simulink library "ROS_lib"  (R2019a)
settings: Solver=VariableStepAuto  StartTime=0.0  StopTime=10.0  RelTol=1e-3
undefined symbols (not defined in the file or in its folder): DiscIntNeverNeededParam
libraries: adeye_lib x26, robotlib x4, PreScanSimulinkLibrary x3
settings Model: Creator=adeye  LastModifiedBy=adeye

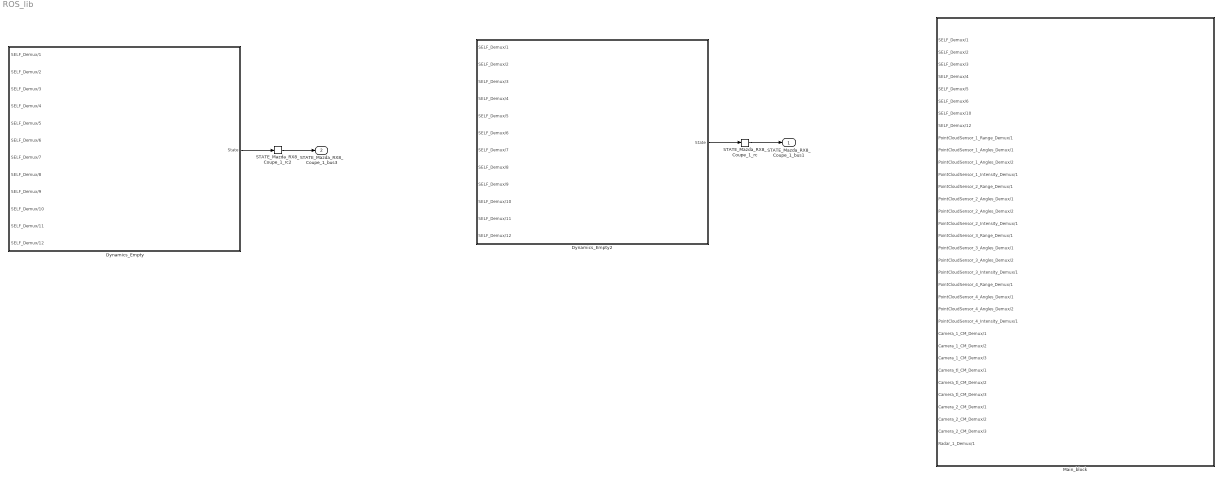
== system ROS_lib ==
  Dynamics_Empty : Subsystem  Tag=Dynamics_Empty
  Dynamics_Empty2 : Subsystem  Tag=Dynamics_Empty
  Main_block : Subsystem
  STATE_Mazda_RX8_Coupe_1_rc : RateTransition  Tag=mux_rc/StatePort  OutPortSampleTimeOpt=Inherit
  STATE_Mazda_RX8_Coupe_1_rc2 : RateTransition  Tag=mux_rc/StatePort  OutPortSampleTimeOpt=Inherit
  STATE_Mazda_RX8_Coupe_1_bus1 : Outport  Tag=outport/StatePort  OutDataTypeStr=Bus: PRESCAN_STATEACTUATORDATA  PortDimensions=1  SampleTime=1/20
  STATE_Mazda_RX8_Coupe_1_bus3 : Outport  Tag=outport/StatePort  Port=2  OutDataTypeStr=Bus: PRESCAN_STATEACTUATORDATA  PortDimensions=1  SampleTime=1/20
  wires:
  STATE_Mazda_RX8_Coupe_1_rc/1 -> STATE_Mazda_RX8_Coupe_1_bus1/1
  Dynamics_Empty2/1(State) -> STATE_Mazda_RX8_Coupe_1_rc/1
  STATE_Mazda_RX8_Coupe_1_rc2/1 -> STATE_Mazda_RX8_Coupe_1_bus3/1
  Dynamics_Empty/1(State) -> STATE_Mazda_RX8_Coupe_1_rc2/1

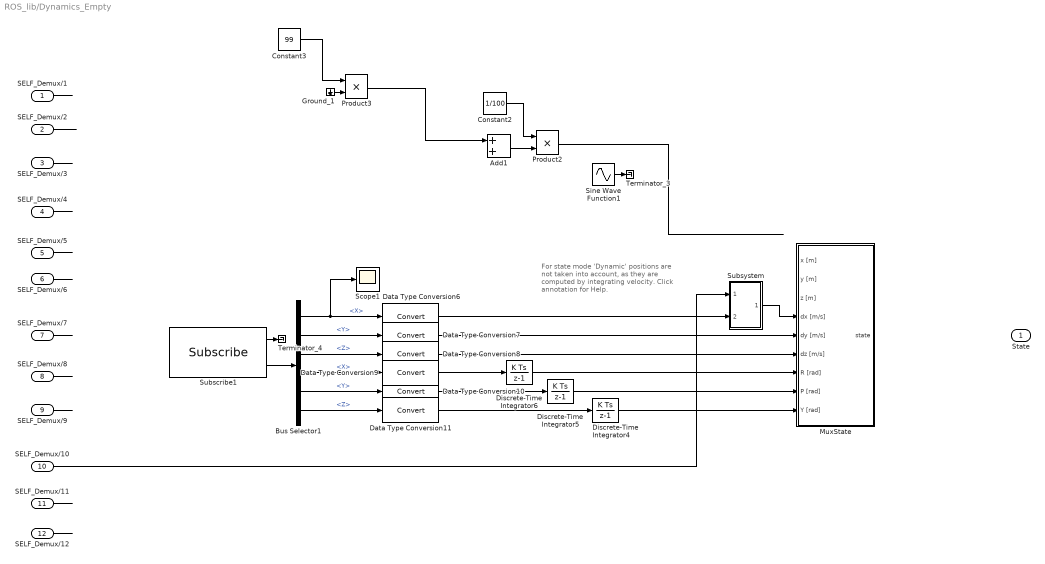
== system ROS_lib/Dynamics_Empty ==
  note: For state mode 'Dynamic' positions
      | are not taken into account, as they
      | are computed by integrating velocity.
      | Click annotation for Help.
  SELF_Demux/1 : Inport
  SELF_Demux/2 : Inport  Port=2
  SELF_Demux/3 : Inport  Port=3
  SELF_Demux/4 : Inport  Port=4
  SELF_Demux/5 : Inport  Port=5
  SELF_Demux/6 : Inport  Port=6
  SELF_Demux/7 : Inport  Port=7
  SELF_Demux/8 : Inport  Port=8
  SELF_Demux/9 : Inport  Port=9
  SELF_Demux/10 : Inport  Port=10
  SELF_Demux/11 : Inport  Port=11
  SELF_Demux/12 : Inport  Port=12
  Add1 : Sum
  Bus Selector1 : BusSelector  OutputSignals=Twist.Linear.X,Twist.Linear.Y,Twist.Linear.Z,Twist.Angular.X,Twist.Angular.Y,Twist.Angular.Z
  Constant2 : Constant  Value=1/100
  Constant3 : Constant  Value=99
  Data Type Conversion{6..11} (6 alike) : DataTypeConversion
  Discrete-Time Integrator4 : DiscreteIntegrator  SampleTime=-1  ICPrevOutput=DiscIntNeverNeededParam  ICPrevScaledInput=DiscIntNeverNeededParam
  Discrete-Time Integrator5 : DiscreteIntegrator  SampleTime=-1  ICPrevOutput=DiscIntNeverNeededParam  ICPrevScaledInput=DiscIntNeverNeededParam
  Discrete-Time Integrator6 : DiscreteIntegrator  SampleTime=-1  ICPrevOutput=DiscIntNeverNeededParam  ICPrevScaledInput=DiscIntNeverNeededParam
  Ground_1 : Ground
  MuxState : Subsystem  Tag=mux/State  mask(Empty Dynamics State Block){positioningmode=off, TimeStep=1/20}
      mask prompts: positioningmode "Positioning Mode"; TimeStep "Auto Assigned: Time Step [s]"
      mask help:
      | Build the state of an actor based on user input.
      | The user can either use positioning mode or dynamics mode.
      | - When using positioning mode the position and orientation of the actor are set directly based on the input. Expected input is relative to the initial position and orientation of the actor. It's also possible to specify the velocity of the actor, though this input isn't used, only passed on.
      | - When using dynamics mode the position input is ignored. Expected input is velocity and orientation. The velocity is relative the current orientation of the actor, while orientation is relative to its initial orientation. The position of the actor is calculated based on the velocity and orientation given.
      settings: DeleteFcn=PreScanBlockDeleteFcn;
  Product2 : Product
  Product3 : Product
  Scope1 : Scope
  Sine Wave Function1 : Sin  Amplitude=0.1  SampleTime=0
  Subscribe1 : robotlib/Subscribe  topicSource=Select from ROS network  topic=/TwistS  messageType=geometry_msgs/TwistStamped  sampleTime=-1  messageQueueLength=1
      settings: SourceProductBaseCode=RO
  Subsystem : Subsystem
  Terminator_3 : Terminator
  Terminator_4 : Terminator
  State : Outport  Tag=outport/StateOutport  SampleTime=1/20
  wires:
  SELF_Demux/1/1 -> ?
  SELF_Demux/2/1 -> ?
  SELF_Demux/12/1 -> ?
  SELF_Demux/6/1 -> ?
  SELF_Demux/11/1 -> ?
  SELF_Demux/8/1 -> ?
  SELF_Demux/9/1 -> ?
  SELF_Demux/7/1 -> ?
  SELF_Demux/4/1 -> ?
  SELF_Demux/3/1 -> ?
  SELF_Demux/5/1 -> ?
  Product2/1 -> ?
  ? -> Add1/2
  Add1/1 -> Product2/2
  Constant2/1 -> Product2/1
  Bus Selector1/5 -> Data Type Conversion10/1  "<Y>"
  Sine Wave Function1/1 -> Terminator_3/1
  Data Type Conversion6/1 -> Subsystem/2(In2)
  Subsystem/1(Out1) -> MuxState/4(dx [m/s])
  Data Type Conversion9/1 -> Discrete-Time Integrator6/1
  Ground_1/1 -> Product3/2
  Subscribe1/1 -> Terminator_4/1
  Subscribe1/2 -> Bus Selector1/1
  Bus Selector1/4 -> Data Type Conversion9/1  "<X>"
  Product3/1 -> Add1/1
  Data Type Conversion11/1 -> Discrete-Time Integrator4/1
  Discrete-Time Integrator4/1 -> MuxState/9(Y [rad])
  Discrete-Time Integrator6/1 -> MuxState/7(R [rad])
  Data Type Conversion8/1 -> MuxState/6(dz [m/s])
  Data Type Conversion10/1 -> Discrete-Time Integrator5/1
  Data Type Conversion7/1 -> MuxState/5(dy [m/s])
  SELF_Demux/10/1 -> Subsystem/1(In1)
  Bus Selector1/1 -> Scope1/1, Data Type Conversion6/1  "<X>"
  Bus Selector1/3 -> Data Type Conversion8/1  "<Z>"
  Discrete-Time Integrator5/1 -> MuxState/8(P [rad])
  Constant3/1 -> Product3/1
  Bus Selector1/6 -> Data Type Conversion11/1  "<Z>"
  Bus Selector1/2 -> Data Type Conversion7/1  "<Y>"

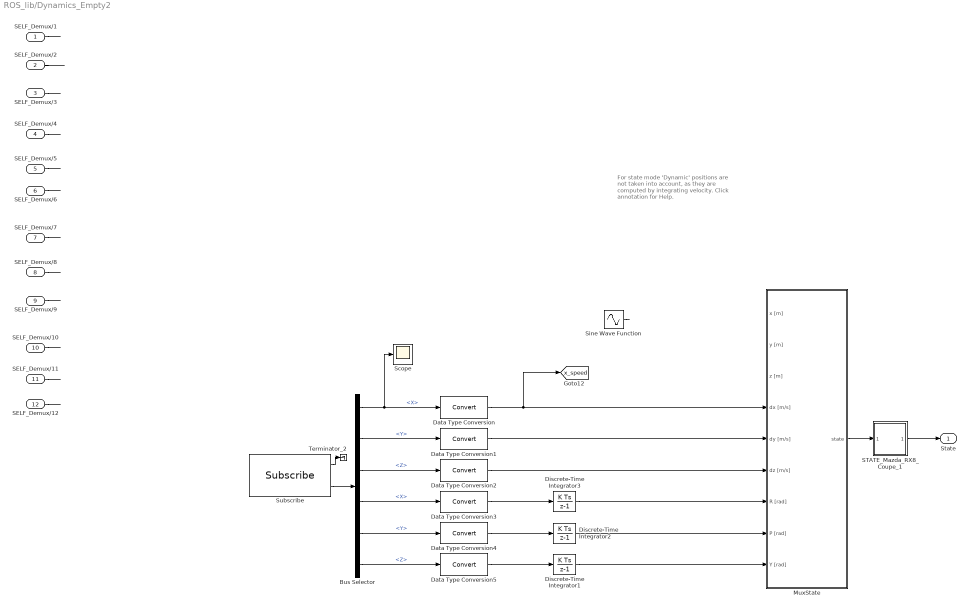
== system ROS_lib/Dynamics_Empty2 ==
  note: For state mode 'Dynamic' positions
      | are not taken into account, as they
      | are computed by integrating velocity.
      | Click annotation for Help.
  SELF_Demux/1 : Inport
  SELF_Demux/2 : Inport  Port=2
  SELF_Demux/3 : Inport  Port=3
  SELF_Demux/4 : Inport  Port=4
  SELF_Demux/5 : Inport  Port=5
  SELF_Demux/6 : Inport  Port=6
  SELF_Demux/7 : Inport  Port=7
  SELF_Demux/8 : Inport  Port=8
  SELF_Demux/9 : Inport  Port=9
  SELF_Demux/10 : Inport  Port=10
  SELF_Demux/11 : Inport  Port=11
  SELF_Demux/12 : Inport  Port=12
  Bus Selector : BusSelector  OutputSignals=Twist.Linear.X,Twist.Linear.Y,Twist.Linear.Z,Twist.Angular.X,Twist.Angular.Y,Twist.Angular.Z
  Data Type Conversion{,1..5} (6 alike) : DataTypeConversion
  Discrete-Time Integrator1 : DiscreteIntegrator  SampleTime=-1  ICPrevOutput=DiscIntNeverNeededParam  ICPrevScaledInput=DiscIntNeverNeededParam
  Discrete-Time Integrator2 : DiscreteIntegrator  SampleTime=-1  ICPrevOutput=DiscIntNeverNeededParam  ICPrevScaledInput=DiscIntNeverNeededParam
  Discrete-Time Integrator3 : DiscreteIntegrator  SampleTime=-1  ICPrevOutput=DiscIntNeverNeededParam  ICPrevScaledInput=DiscIntNeverNeededParam
  MuxState : Subsystem  Tag=mux/State  mask(Empty Dynamics State Block){positioningmode=off, TimeStep=1/20}
      mask prompts: positioningmode "Positioning Mode"; TimeStep "Auto Assigned: Time Step [s]"
      mask help:
      | Build the state of an actor based on user input.
      | The user can either use positioning mode or dynamics mode.
      | - When using positioning mode the position and orientation of the actor are set directly based on the input. Expected input is relative to the initial position and orientation of the actor. It's also possible to specify the velocity of the actor, though this input isn't used, only passed on.
      | - When using dynamics mode the position input is ignored. Expected input is velocity and orientation. The velocity is relative the current orientation of the actor, while orientation is relative to its initial orientation. The position of the actor is calculated based on the velocity and orientation given.
      settings: DeleteFcn=PreScanBlockDeleteFcn;
  STATE_Mazda_RX8_Coupe_1 : Subsystem  Tag=mux/StatePort  Priority=0  LoadFcn=load PrescanStateActuatorData  mask(PreScan Sink Block: State){x0=74.1475, y0=27.5553, z0=0.51, Roll0=0, Pitch0=0, Yaw0=0, TimeStep=1/20}
      mask prompts: x0 "Ini x-position VEHICLE wrt GLOBAL axis system [m]"; y0 "Ini y-position VEHICLE wrt GLOBAL axis system [m]"; z0 "Ini z-position VEHICLE wrt GLOBAL axis system [m]"; Roll0 "Ini roll-angle BODY wrt VEHICLE axis system [deg]"; Pitch0 "Ini pitch-angle BODY wrt VEHICLE axis system [deg]"; Yaw0 "Ini yaw-angle VEHICLE wrt GLOBAL axis system [deg]"; TimeStep "Auto-Assigned: Upload Period [s]"
      mask help:
      | The Actor State contains a vector signal of size (9x1), containing the following signals:
      |
      | -  Position                  (x,y,z)                                     [m]
      | -  Velocity                  (vx,vy,vz)                               [m/s]
      | -  Angles                    (Roll, Pitch, Yaw)                   [rad]
      |
      | The Actor state is defined in the global axis system.
      | The state is superponed on the Initial position defined in the GUI.
      |
      | For more information, please click Help.
      settings: DeleteFcn=PreScanBlockDeleteFcn;
      mask Help: eval('openHelp(222)')
      mask Display: image(imread('State.png'))
  Scope : Scope
  Sine Wave Function : Sin  Amplitude=0.1  SampleTime=0
  Subscribe : robotlib/Subscribe  topicSource=Select from ROS network  topic=/TwistS  messageType=geometry_msgs/TwistStamped  sampleTime=-1  messageQueueLength=1
      settings: SourceProductBaseCode=RO
  Terminator_2 : Terminator
  State : Outport  Tag=outport/StateOutport  SampleTime=1/20
  tag scope: x_speed=global
  wires:
  Bus Selector/1 -> Scope/1, Data Type Conversion/1  "<X>"
  Data Type Conversion/1 -> [x_speed], MuxState/4(dx [m/s])
  Bus Selector/2 -> Data Type Conversion1/1  "<Y>"
  Bus Selector/3 -> Data Type Conversion2/1  "<Z>"
  Bus Selector/4 -> Data Type Conversion3/1  "<X>"
  Data Type Conversion3/1 -> Discrete-Time Integrator3/1
  Bus Selector/5 -> Data Type Conversion4/1  "<Y>"
  Data Type Conversion4/1 -> Discrete-Time Integrator2/1
  Bus Selector/6 -> Data Type Conversion5/1  "<Z>"
  Data Type Conversion5/1 -> Discrete-Time Integrator1/1
  Subscribe/2 -> Bus Selector/1
  Data Type Conversion1/1 -> MuxState/5(dy [m/s])
  Data Type Conversion2/1 -> MuxState/6(dz [m/s])
  Discrete-Time Integrator3/1 -> MuxState/7(R [rad])
  Discrete-Time Integrator2/1 -> MuxState/8(P [rad])
  Discrete-Time Integrator1/1 -> MuxState/9(Y [rad])
  Sine Wave Function/1 -> ?
  Subscribe/1 -> Terminator_2/1
  MuxState/1(state) -> STATE_Mazda_RX8_Coupe_1/1(State)
  STATE_Mazda_RX8_Coupe_1/1(StateBus) -> State/1
  SELF_Demux/1/1 -> ?
  SELF_Demux/2/1 -> ?
  SELF_Demux/12/1 -> ?
  SELF_Demux/6/1 -> ?
  SELF_Demux/11/1 -> ?
  SELF_Demux/8/1 -> ?
  SELF_Demux/9/1 -> ?
  SELF_Demux/7/1 -> ?
  SELF_Demux/4/1 -> ?
  SELF_Demux/10/1 -> ?
  SELF_Demux/3/1 -> ?
  SELF_Demux/5/1 -> ?

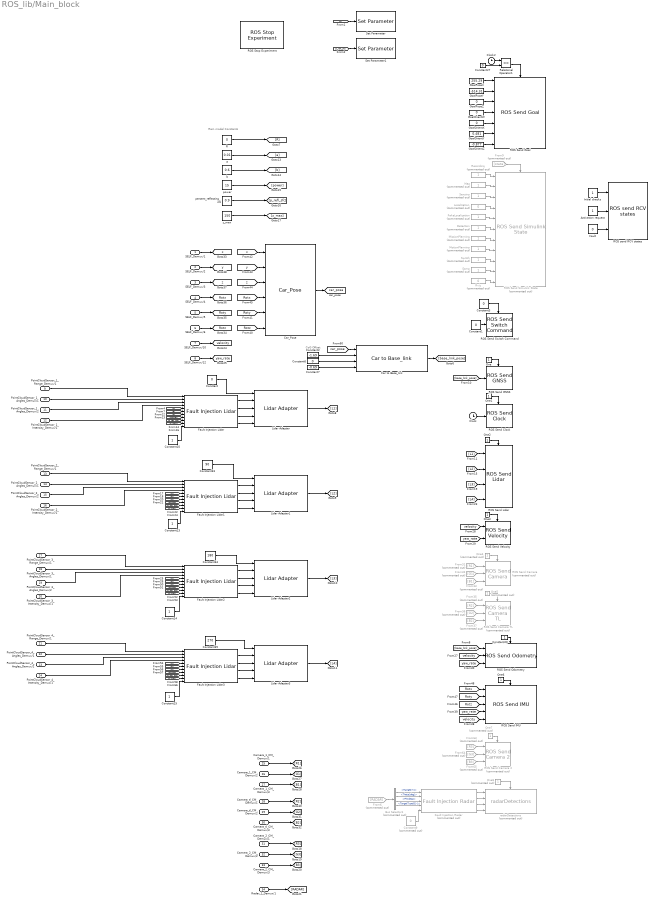
== system ROS_lib/Main_block ==
  note: Rain model Constants
  note: CoG Offset
  SELF_Demux/1 : Inport
  SELF_Demux/2 : Inport  Port=2
  SELF_Demux/3 : Inport  Port=3
  SELF_Demux/4 : Inport  Port=4
  SELF_Demux/5 : Inport  Port=5
  SELF_Demux/6 : Inport  Port=6
  SELF_Demux/10 : Inport  Port=7
  SELF_Demux/12 : Inport  Port=8
  PointCloudSensor_1_Range_Demux/1 : Inport  Port=9
  PointCloudSensor_1_Angles_Demux/1 : Inport  Port=10
  PointCloudSensor_1_Angles_Demux/2 : Inport  Port=11
  PointCloudSensor_1_Intensity_Demux/1 : Inport  Port=12
  PointCloudSensor_2_Range_Demux/1 : Inport  Port=13
  PointCloudSensor_2_Angles_Demux/1 : Inport  Port=14
  PointCloudSensor_2_Angles_Demux/2 : Inport  Port=15
  PointCloudSensor_2_Intensity_Demux/1 : Inport  Port=16
  PointCloudSensor_3_Range_Demux/1 : Inport  Port=17
  PointCloudSensor_3_Angles_Demux/1 : Inport  Port=18
  PointCloudSensor_3_Angles_Demux/2 : Inport  Port=19
  PointCloudSensor_3_Intensity_Demux/1 : Inport  Port=20
  PointCloudSensor_4_Range_Demux/1 : Inport  Port=21
  PointCloudSensor_4_Angles_Demux/1 : Inport  Port=22
  PointCloudSensor_4_Angles_Demux/2 : Inport  Port=23
  PointCloudSensor_4_Intensity_Demux/1 : Inport  Port=24
  Camera_1_CM_Demux/1 : Inport  Port=25
  Camera_1_CM_Demux/2 : Inport  Port=26
  Camera_1_CM_Demux/3 : Inport  Port=27
  Camera_tl_CM_Demux/1 : Inport  Port=28
  Camera_tl_CM_Demux/2 : Inport  Port=29
  Camera_tl_CM_Demux/3 : Inport  Port=30
  Camera_2_CM_Demux/1 : Inport  Port=31
  Camera_2_CM_Demux/2 : Inport  Port=32
  Camera_2_CM_Demux/3 : Inport  Port=33
  Radar_1_Demux/1 : Inport  Port=34
  Activation request : Constant  OutDataTypeStr=Inherit: Inherit via back propagation
  Bus Selector1 : BusSelector  Commented=on  OutputSignals=Range[m],Theta[deg],Phi[deg],TargetTypeID[-]
  Car to Base_link : adeye_lib/Car to Base_link  SystemSampleTime=-1
  Car_Pose : adeye_lib/Car_Pose  SystemSampleTime=-1
  Clock : Clock
  Clock2 : Clock
  Constant : Constant  Value=0  OutDataTypeStr=Inherit: Inherit via back propagation
  Constant1 : Constant  Value=0  OutDataTypeStr=int32
  Constant{10,13..15} (4 alike) : Constant  OutDataTypeStr=Inherit: Inherit via back propagation
  Constant2 : Constant  Value=-1.69
  Constant20 : Constant
  Constant27 : Constant  Value=0
  Constant3 : Constant  Value=0
  Constant33 : Constant  Value=90  OutDataTypeStr=Inherit: Inherit via back propagation
  Constant34 : Constant  Value=180  OutDataTypeStr=Inherit: Inherit via back propagation
  Constant35 : Constant  Value=270  OutDataTypeStr=Inherit: Inherit via back propagation
  Constant6 : Constant  Value=0
  Constant7 : Constant  Value=-0.69
  Constant9 : Constant  Commented=on  Value=0
  Detection : Constant  Commented=on
  FakeLocalization : Constant  Commented=on
  Fault : Constant  Value=0  OutDataTypeStr=Inherit: Inherit via back propagation
  Fault Injection Lidar{,1..3} (4 alike) : adeye_lib/Fault Injection Lidar  vr=0.0001  vi=0.0001  f=20  p=225*16
  Fault Injection Radar : adeye_lib/Fault Injection Radar  Commented=on  n=7  vr=1  vt=1  vp=1
  From31 : From  Commented=on  GotoTag=R1
  From32 : From  Commented=on  GotoTag=G1
  From33 : From  Commented=on  GotoTag=B1
  From35 : From  Commented=on  GotoTag=R2
  From36 : From  Commented=on  GotoTag=G2
  From37 : From  Commented=on  GotoTag=B2
  From6 : From  Commented=on  GotoTag=RADAR
  From63 : From  Commented=on  GotoTag=R3
  From64 : From  Commented=on  GotoTag=G3
  From65 : From  Commented=on  GotoTag=B3
  From9 : From  Commented=on  GotoTag=state
  GoalOrientW : Constant  Value=0
  GoalOrientX : Constant  Value=0
  GoalOrientY : Constant  Value=0.481
  GoalOrientZ : Constant  Value=-0.877
  GoalPoseX : Constant  Value=255.29
  GoalPoseY : Constant  Value=-514.31
  GoalPoseZ : Constant  Value=0
  Initial checks : Constant  OutDataTypeStr=Inherit: Inherit via back propagation
  Lidar Adapter{,1..3} (4 alike) : adeye_lib/Lidar Adapter  SystemSampleTime=-1
  Localization : Constant  Commented=on  Value=0
  Map : Constant  Commented=on
  MissionPlanning : Constant  Commented=on
  MotionPlanning : Constant  Commented=on
  One{,1..3,6} (5 alike) : Constant  OutDataTypeStr=Inherit: Inherit via back propagation
  One{4..5,7..8} (4 alike) : Constant  Commented=on  OutDataTypeStr=Inherit: Inherit via back propagation
  R : Constant  Value=0
  ROS Send Camera : adeye_lib/ROS Send Camera  Commented=on  SystemSampleTime=-1
  ROS Send Camera 2 : adeye_lib/ROS Send Camera 2  Commented=on  SystemSampleTime=-1
  ROS Send Camera TL : adeye_lib/ROS Send Camera TL  Commented=on  SystemSampleTime=-1
  ROS Send Clock : adeye_lib/ROS Send Clock  SystemSampleTime=-1
  ROS Send GNSS : adeye_lib/ROS Send GNSS  SystemSampleTime=-1
  ROS Send Goal : adeye_lib/ROS Send Goal  SystemSampleTime=-1
  ROS Send IMU : adeye_lib/ROS Send IMU  SystemSampleTime=-1
  ROS Send Lidar : adeye_lib/ROS Send Lidar  SystemSampleTime=-1
  ROS Send Odometry : adeye_lib/ROS Send Odometry  SystemSampleTime=-1
  ROS Send Simulink State : adeye_lib/ROS Send Simulink State  Commented=on  SystemSampleTime=-1
  ROS Send Switch Command : adeye_lib/ROS Send Switch Command  SystemSampleTime=-1
  ROS Send Velocity : adeye_lib/ROS Send Velocity  SystemSampleTime=-1
  ROS Stop Experiment : adeye_lib/ROS Stop Experiment  SystemSampleTime=-1
  ROS send RCV states : adeye_lib/ROS send RCV states  SystemSampleTime=-1
  Recording : Constant  Commented=on
  Relational Operator1 : RelationalOperator  Operator===  OutDataTypeStr=boolean  RndMeth=Simplest
  Rviz : Constant  Commented=on  Value=0
  Sensing : Constant  Commented=on
  Set Parameter : robotlib/Set Parameter  ParameterSource=Specify your own  ParameterName=/simulink/rain_intensity  ParameterType=double  ModelName=ROS_lib  BlockId=ParamSet_ROS_lib_3479
      settings: SourceProductName=Robotics System Toolbox  SourceProductBaseCode=RO
  Set Parameter1 : robotlib/Set Parameter  ParameterSource=Specify your own  ParameterName=/simulink/reflectivity  ParameterType=double  ModelName=ROS_lib  BlockId=ParamSet_ROS_lib_3480
      settings: SourceProductName=Robotics System Toolbox  SourceProductBaseCode=RO
  Ssmp : Constant  Commented=on
  Switch : Constant  Commented=on
  a : Constant  Value=0.01
  b : Constant  Value=0.6
  percent_reflecting_sfc : Constant  Value=0.9
  power : Constant  Value=15
  radarDetections : adeye_lib/radarDetections  Commented=on  SystemSampleTime=-1
  z_max : Constant  Value=150
  tag scope: Rotx=global, Roty=global, Rotz=global, car_pose=global, velocity=global, x=global, y=global, yaw_rate=global, z=global
  wires:
  [velocity] -> ROS Send Odometry/2
  [yaw_rate] -> ROS Send Odometry/3
  [Rotx] -> ROS Send IMU/1
  Relational Operator1/1 -> ROS Send Goal/Enable
  Clock2/1 -> Relational Operator1/1
  [base_link_pose] -> ROS Send Odometry/1
  One1/1 -> ROS Send Clock/Enable
  From36/1 -> ROS Send Camera TL/2
  [L1] -> ROS Send Lidar/1
  [L2] -> ROS Send Lidar/2
  [yaw_rate] -> ROS Send IMU/4
  From33/1 -> ROS Send Camera/3
  One/1 -> ROS Send GNSS/Enable
  [L3] -> ROS Send Lidar/3
  Constant27/1 -> Relational Operator1/2
  [Rotz] -> ROS Send IMU/3
  [velocity] -> ROS Send Velocity/1
  [yaw_rate] -> ROS Send Velocity/2
  [Roty] -> ROS Send IMU/2
  From37/1 -> ROS Send Camera TL/3
  Clock/1 -> ROS Send Clock/1
  [base_link_pose] -> ROS Send GNSS/1
  [velocity] -> ROS Send IMU/5
  From31/1 -> ROS Send Camera/1
  From32/1 -> ROS Send Camera/2
  [L4] -> ROS Send Lidar/4
  From35/1 -> ROS Send Camera TL/1
  Constant20/1 -> ROS Send Odometry/Enable
  Camera_tl_CM_Demux/1/1 -> [R2]
  Camera_1_CM_Demux/3/1 -> [B1]
  Camera_tl_CM_Demux/2/1 -> [G2]
  Camera_tl_CM_Demux/3/1 -> [B2]
  Camera_1_CM_Demux/2/1 -> [G1]
  Camera_1_CM_Demux/1/1 -> [R1]
  SELF_Demux/3/1 -> [z]
  SELF_Demux/2/1 -> [y]
  [Rotz] -> Car_Pose/6
  SELF_Demux/6/1 -> [Rotz]
  Car_Pose/1 -> [car_pose]
  SELF_Demux/1/1 -> [x]
  SELF_Demux/4/1 -> [Rotx]
  [z] -> Car_Pose/3
  SELF_Demux/12/1 -> [yaw_rate]
  [Rotx] -> Car_Pose/4
  [y] -> Car_Pose/2
  SELF_Demux/5/1 -> [Roty]
  SELF_Demux/10/1 -> [velocity]
  [x] -> Car_Pose/1
  [Roty] -> Car_Pose/5
  power/1 -> [power]
  percent_reflecting_sfc/1 -> [p_refl_sfc]
  b/1 -> [b]
  a/1 -> [a]
  R/1 -> [R]
  z_max/1 -> [z_max]
  [car_pose] -> Car to Base_link/1
  Constant2/1 -> Car to Base_link/2
  Constant7/1 -> Car to Base_link/4
  Car to Base_link/1 -> [base_link_pose]
  Constant6/1 -> Car to Base_link/3
  GoalPoseX/1 -> ROS Send Goal/1
  GoalPoseY/1 -> ROS Send Goal/2
  GoalPoseZ/1 -> ROS Send Goal/3
  GoalOrientW/1 -> ROS Send Goal/4
  GoalOrientX/1 -> ROS Send Goal/5
  GoalOrientY/1 -> ROS Send Goal/6
  GoalOrientZ/1 -> ROS Send Goal/7
  Constant1/1 -> ROS Send Switch Command/1
  Constant3/1 -> ROS Send Switch Command/Enable
  Camera_2_CM_Demux/1/1 -> [R3]
  Camera_2_CM_Demux/2/1 -> [G3]
  Camera_2_CM_Demux/3/1 -> [B3]
  Radar_1_Demux/1/1 -> [RADAR]
  Fault Injection Radar/2 -> radarDetections/2
  Bus Selector1/4 -> Fault Injection Radar/4  "<TargetTypeID[-]>"
  Constant9/1 -> Fault Injection Radar/5
  Fault Injection Radar/1 -> radarDetections/1
  Fault Injection Radar/3 -> radarDetections/3
  Bus Selector1/2 -> Fault Injection Radar/2  "<Theta[deg]>"
  From6/1 -> Bus Selector1/1
  Fault Injection Radar/4 -> radarDetections/4
  Bus Selector1/1 -> Fault Injection Radar/1  "<Range[m]>"
  Bus Selector1/3 -> Fault Injection Radar/3  "<Phi[deg]>"
  From64/1 -> ROS Send Camera 2/2
  From65/1 -> ROS Send Camera 2/3
  From63/1 -> ROS Send Camera 2/1
  Lidar Adapter/1 -> [L1]
  Constant/1 -> Lidar Adapter/1
  Fault Injection Lidar/4 -> Lidar Adapter/5
  Fault Injection Lidar/1 -> Lidar Adapter/2
  Fault Injection Lidar/2 -> Lidar Adapter/3
  Fault Injection Lidar/3 -> Lidar Adapter/4
  Constant10/1 -> Fault Injection Lidar/11
  [p_refl_sfc] -> Fault Injection Lidar/9
  [a] -> Fault Injection Lidar/6
  [z_max] -> Fault Injection Lidar/10
  [power] -> Fault Injection Lidar/8
  [b] -> Fault Injection Lidar/7
  [R] -> Fault Injection Lidar/5
  PointCloudSensor_1_Range_Demux/1/1 -> Fault Injection Lidar/1
  PointCloudSensor_1_Angles_Demux/1/1 -> Fault Injection Lidar/2
  PointCloudSensor_1_Angles_Demux/2/1 -> Fault Injection Lidar/3
  PointCloudSensor_1_Intensity_Demux/1/1 -> Fault Injection Lidar/4
  Constant33/1 -> Lidar Adapter1/1
  Lidar Adapter1/1 -> [L2]
  [power] -> Fault Injection Lidar1/8
  [z_max] -> Fault Injection Lidar1/10
  [R] -> Fault Injection Lidar1/5
  [a] -> Fault Injection Lidar1/6
  Fault Injection Lidar1/1 -> Lidar Adapter1/2
  Fault Injection Lidar1/3 -> Lidar Adapter1/4
  Constant13/1 -> Fault Injection Lidar1/11
  Fault Injection Lidar1/4 -> Lidar Adapter1/5
  [p_refl_sfc] -> Fault Injection Lidar1/9
  [b] -> Fault Injection Lidar1/7
  Fault Injection Lidar1/2 -> Lidar Adapter1/3
  PointCloudSensor_2_Range_Demux/1/1 -> Fault Injection Lidar1/1
  PointCloudSensor_2_Angles_Demux/1/1 -> Fault Injection Lidar1/2
  PointCloudSensor_2_Angles_Demux/2/1 -> Fault Injection Lidar1/3
  PointCloudSensor_2_Intensity_Demux/1/1 -> Fault Injection Lidar1/4
  [z_max] -> Fault Injection Lidar2/10
  [power] -> Fault Injection Lidar2/8
  [p_refl_sfc] -> Fault Injection Lidar2/9
  [R] -> Fault Injection Lidar2/5
  Constant14/1 -> Fault Injection Lidar2/11
  [a] -> Fault Injection Lidar2/6
  Fault Injection Lidar2/1 -> Lidar Adapter2/2
  Lidar Adapter2/1 -> [L3]
  Fault Injection Lidar2/3 -> Lidar Adapter2/4
  Fault Injection Lidar2/4 -> Lidar Adapter2/5
  Constant34/1 -> Lidar Adapter2/1
  Fault Injection Lidar2/2 -> Lidar Adapter2/3
  [b] -> Fault Injection Lidar2/7
  PointCloudSensor_3_Range_Demux/1/1 -> Fault Injection Lidar2/1
  PointCloudSensor_3_Angles_Demux/1/1 -> Fault Injection Lidar2/2
  PointCloudSensor_3_Angles_Demux/2/1 -> Fault Injection Lidar2/3
  PointCloudSensor_3_Intensity_Demux/1/1 -> Fault Injection Lidar2/4
  [a] -> Fault Injection Lidar3/6
  Fault Injection Lidar3/3 -> Lidar Adapter3/4
  Fault Injection Lidar3/1 -> Lidar Adapter3/2
  [p_refl_sfc] -> Fault Injection Lidar3/9
  [b] -> Fault Injection Lidar3/7
  [z_max] -> Fault Injection Lidar3/10
  Constant35/1 -> Lidar Adapter3/1
  Fault Injection Lidar3/2 -> Lidar Adapter3/3
  Lidar Adapter3/1 -> [L4]
  Constant15/1 -> Fault Injection Lidar3/11
  [power] -> Fault Injection Lidar3/8
  Fault Injection Lidar3/4 -> Lidar Adapter3/5
  [R] -> Fault Injection Lidar3/5
  PointCloudSensor_4_Range_Demux/1/1 -> Fault Injection Lidar3/1
  PointCloudSensor_4_Angles_Demux/1/1 -> Fault Injection Lidar3/2
  PointCloudSensor_4_Angles_Demux/2/1 -> Fault Injection Lidar3/3
  PointCloudSensor_4_Intensity_Demux/1/1 -> Fault Injection Lidar3/4
  Fault/1 -> ROS send RCV states/3
  Initial checks/1 -> ROS send RCV states/1
  Activation request/1 -> ROS send RCV states/2
  Rviz/1 -> ROS Send Simulink State/11
  Switch/1 -> ROS Send Simulink State/9
  Localization/1 -> ROS Send Simulink State/4
  Detection/1 -> ROS Send Simulink State/6
  From9/1 -> ROS Send Simulink State/Enable
  FakeLocalization/1 -> ROS Send Simulink State/5
  Recording/1 -> ROS Send Simulink State/1
  MotionPlanning/1 -> ROS Send Simulink State/8
  Map/1 -> ROS Send Simulink State/2
  MissionPlanning/1 -> ROS Send Simulink State/7
  Ssmp/1 -> ROS Send Simulink State/10
  Sensing/1 -> ROS Send Simulink State/3
  One2/1 -> ROS Send Lidar/Enable
  One3/1 -> ROS Send Velocity/Enable
  One4/1 -> ROS Send Camera/Enable
  One5/1 -> ROS Send Camera TL/Enable
  One6/1 -> ROS Send IMU/Enable
  One7/1 -> ROS Send Camera 2/Enable
  One8/1 -> radarDetections/Enable
  [R] -> Set Parameter/1
  [p_refl_sfc] -> Set Parameter1/1

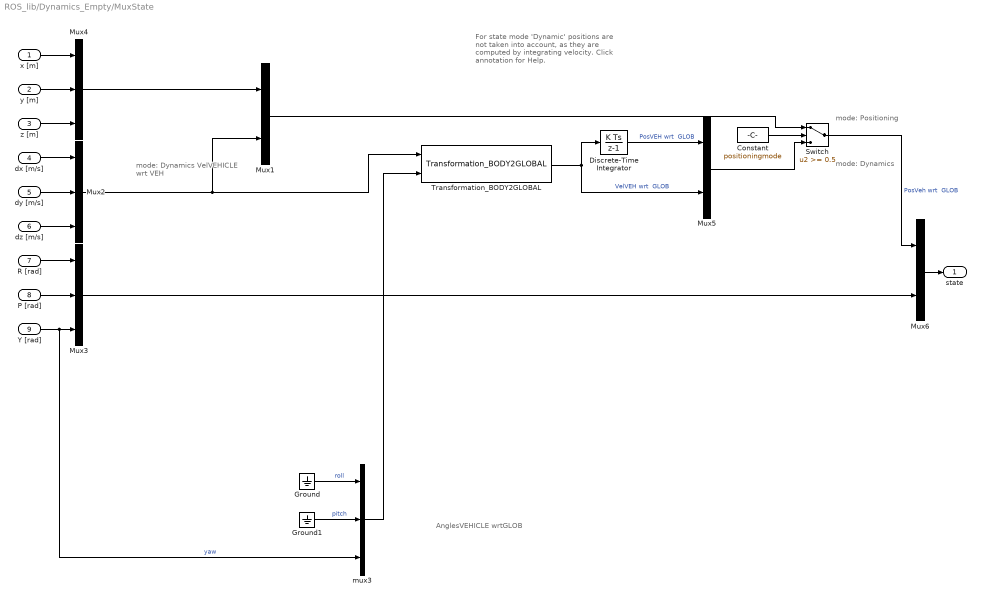
== system ROS_lib/Dynamics_Empty/MuxState ==
  note: mode: Dynamics
  note: mode: Positioning
  note: mode: Dynamics
      | VelVEHICLE
      | wrt VEH
  note: AnglesVEHICLE
      | wrtGLOB
  note: For state mode 'Dynamic' positions
      | are not taken into account, as they
      | are computed by integrating velocity.
      | Click annotation for Help.
  x [m] : Inport  SampleTime=TimeStep
  y [m] : Inport  Port=2  SampleTime=TimeStep
  z [m] : Inport  Port=3  SampleTime=TimeStep
  dx [m/s] : Inport  Port=4  SampleTime=TimeStep
  dy [m/s] : Inport  Port=5  SampleTime=TimeStep
  dz [m/s] : Inport  Port=6  SampleTime=TimeStep
  R [rad] : Inport  Port=7  SampleTime=TimeStep
  P [rad] : Inport  Port=8  SampleTime=TimeStep
  Y [rad] : Inport  Port=9  SampleTime=TimeStep
  Constant : Constant  DisableCoverage=on  Value=positioningmode
  Discrete-Time Integrator : DiscreteIntegrator  SampleTime=TimeStep  ICPrevOutput=DiscIntNeverNeededParam  ICPrevScaledInput=DiscIntNeverNeededParam
  Ground : Ground
  Ground1 : Ground
  Mux1 : Mux  Inputs=[3 3]
  Mux2 : Mux  Inputs=3
  Mux3 : Mux  Inputs=3
  Mux4 : Mux  Inputs=3
  Mux5 : Mux  Inputs=[3 3]
  Mux6 : Mux  Inputs=[6 3]
  Switch : Switch  Threshold=0.5
  Transformation_BODY2GLOBAL : PreScanSimulinkLibrary/Simple_Vehicle_Dynamics/Chassis/MuxDynState/Transformation_BODY2GLOBAL  SystemSampleTime=-1
  mux3 : Mux  Inputs=3
  state : Outport
  wires:
  Constant/1 -> Switch/2
  Mux6/1 -> state/1
  Mux4/1 -> Mux1/1
  Mux5/1 -> Switch/3
  Mux1/1 -> Switch/1
  Switch/1 -> Mux6/1  "PosVeh wrt  GLOB"
  P [rad]/1 -> Mux3/2
  R [rad]/1 -> Mux3/1
  dz [m/s]/1 -> Mux2/3
  dy [m/s]/1 -> Mux2/2
  dx [m/s]/1 -> Mux2/1
  z [m]/1 -> Mux4/3
  y [m]/1 -> Mux4/2
  x [m]/1 -> Mux4/1
  Ground1/1 -> mux3/2  "pitch"
  Y [rad]/1 -> mux3/3, Mux3/3  "yaw"
  Mux3/1 -> Mux6/2
  Transformation_BODY2GLOBAL/1 -> Discrete-Time Integrator/1, Mux5/2  "VelVEH wrt  GLOB"
  mux3/1 -> Transformation_BODY2GLOBAL/2
  Ground/1 -> mux3/1  "roll"
  Mux2/1 -> Mux1/2, Transformation_BODY2GLOBAL/1
  Discrete-Time Integrator/1 -> Mux5/1  "PosVEH wrt  GLOB"

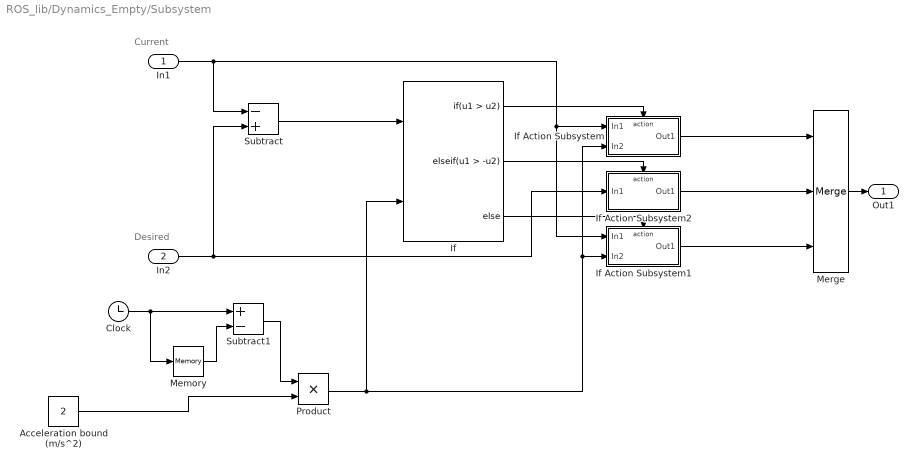
== system ROS_lib/Dynamics_Empty/Subsystem ==
  note: Desired
  note: Current
  In1 : Inport
  In2 : Inport  Port=2
  Acceleration bound (m/s^2) : Constant  Value=2
  Clock : Clock
  If : If  NumInputs=2  IfExpression=u1 > u2  ElseIfExpressions=u1 > -u2
  If Action Subsystem : Subsystem  TreatAsAtomicUnit=on
  If Action Subsystem1 : Subsystem  TreatAsAtomicUnit=on
  If Action Subsystem2 : Subsystem  TreatAsAtomicUnit=on
  Memory : Memory
  Merge : Merge  Inputs=3
  Product : Product
  Subtract : Sum  Inputs=-+
  Subtract1 : Sum  Inputs=+-
  Out1 : Outport
  wires:
  If Action Subsystem/1(Out1) -> Merge/1
  If/3 -> If Action Subsystem1/Action
  Merge/1 -> Out1/1
  If Action Subsystem2/1(Out1) -> Merge/2
  If/2 -> If Action Subsystem2/Action
  If/1 -> If Action Subsystem/Action
  If Action Subsystem1/1(Out1) -> Merge/3
  In1/1 -> If Action Subsystem1/1(In1), If Action Subsystem/1(In1), Subtract/1
  In2/1 -> Subtract/2, If Action Subsystem2/1(In1)
  Subtract/1 -> If/1
  Subtract1/1 -> Product/1
  Product/1 -> If/2, If Action Subsystem1/2(In2), If Action Subsystem/2(In2)
  Acceleration bound (m/s^2)/1 -> Product/2
  Clock/1 -> Memory/1, Subtract1/1
  Memory/1 -> Subtract1/2

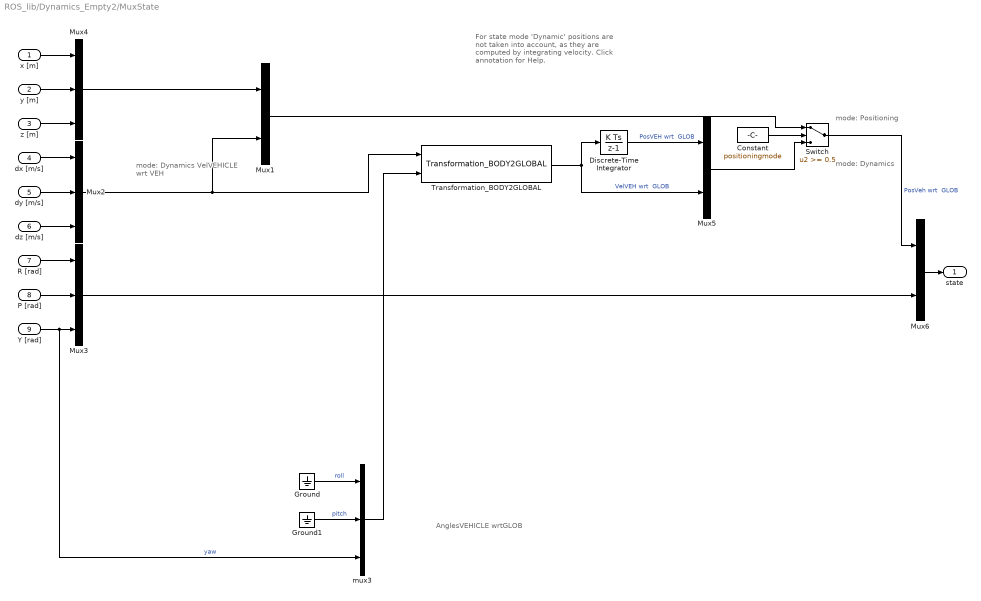
== system ROS_lib/Dynamics_Empty2/MuxState ==
  note: mode: Dynamics
  note: mode: Positioning
  note: mode: Dynamics
      | VelVEHICLE
      | wrt VEH
  note: AnglesVEHICLE
      | wrtGLOB
  note: For state mode 'Dynamic' positions
      | are not taken into account, as they
      | are computed by integrating velocity.
      | Click annotation for Help.
  x [m] : Inport  SampleTime=TimeStep
  y [m] : Inport  Port=2  SampleTime=TimeStep
  z [m] : Inport  Port=3  SampleTime=TimeStep
  dx [m/s] : Inport  Port=4  SampleTime=TimeStep
  dy [m/s] : Inport  Port=5  SampleTime=TimeStep
  dz [m/s] : Inport  Port=6  SampleTime=TimeStep
  R [rad] : Inport  Port=7  SampleTime=TimeStep
  P [rad] : Inport  Port=8  SampleTime=TimeStep
  Y [rad] : Inport  Port=9  SampleTime=TimeStep
  Constant : Constant  DisableCoverage=on  Value=positioningmode
  Discrete-Time Integrator : DiscreteIntegrator  SampleTime=TimeStep  ICPrevOutput=DiscIntNeverNeededParam  ICPrevScaledInput=DiscIntNeverNeededParam
  Ground : Ground
  Ground1 : Ground
  Mux1 : Mux  Inputs=[3 3]
  Mux2 : Mux  Inputs=3
  Mux3 : Mux  Inputs=3
  Mux4 : Mux  Inputs=3
  Mux5 : Mux  Inputs=[3 3]
  Mux6 : Mux  Inputs=[6 3]
  Switch : Switch  Threshold=0.5
  Transformation_BODY2GLOBAL : PreScanSimulinkLibrary/Simple_Vehicle_Dynamics/Chassis/MuxDynState/Transformation_BODY2GLOBAL  SystemSampleTime=-1
  mux3 : Mux  Inputs=3
  state : Outport
  wires:
  Constant/1 -> Switch/2
  Mux6/1 -> state/1
  Mux4/1 -> Mux1/1
  Mux5/1 -> Switch/3
  Mux1/1 -> Switch/1
  Switch/1 -> Mux6/1  "PosVeh wrt  GLOB"
  P [rad]/1 -> Mux3/2
  R [rad]/1 -> Mux3/1
  dz [m/s]/1 -> Mux2/3
  dy [m/s]/1 -> Mux2/2
  dx [m/s]/1 -> Mux2/1
  z [m]/1 -> Mux4/3
  y [m]/1 -> Mux4/2
  x [m]/1 -> Mux4/1
  Ground1/1 -> mux3/2  "pitch"
  Y [rad]/1 -> mux3/3, Mux3/3  "yaw"
  Mux3/1 -> Mux6/2
  Transformation_BODY2GLOBAL/1 -> Discrete-Time Integrator/1, Mux5/2  "VelVEH wrt  GLOB"
  mux3/1 -> Transformation_BODY2GLOBAL/2
  Ground/1 -> mux3/1  "roll"
  Mux2/1 -> Mux1/2, Transformation_BODY2GLOBAL/1
  Discrete-Time Integrator/1 -> Mux5/1  "PosVEH wrt  GLOB"

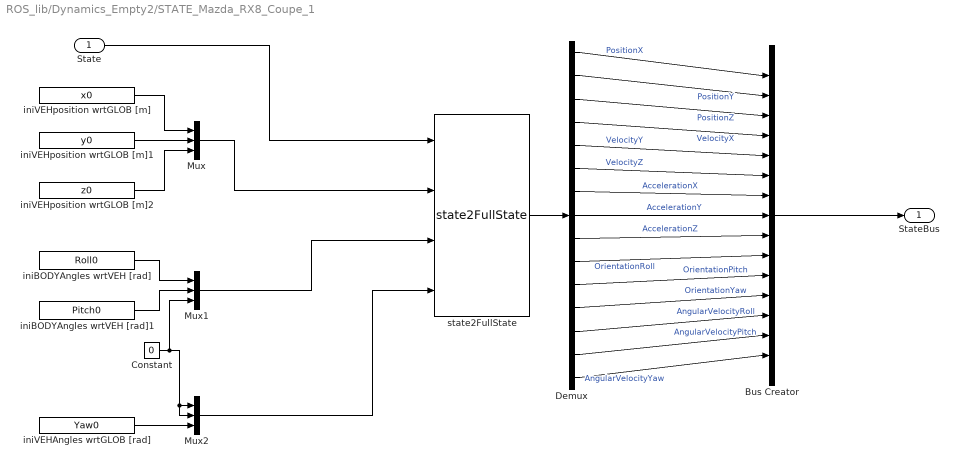
== system ROS_lib/Dynamics_Empty2/STATE_Mazda_RX8_Coupe_1 ==
  State : Inport  SampleTime=TimeStep
  Bus Creator : BusCreator  Inputs=15  OutDataTypeStr=Bus: PRESCAN_STATEACTUATORDATA  NonVirtualBus=on
  Constant : Constant  Value=0
  Demux : Demux  Outputs=15
  Mux : Mux  Inputs=3
  Mux1 : Mux  Inputs=3
  Mux2 : Mux  Inputs=3
  iniBODYAngles wrtVEH [rad] : Constant  Value=Roll0  SampleTime=TimeStep
  iniBODYAngles wrtVEH [rad]1 : Constant  Value=Pitch0  SampleTime=TimeStep
  iniVEHAngles wrtGLOB [rad] : Constant  Value=Yaw0  SampleTime=TimeStep
  iniVEHposition wrtGLOB [m] : Constant  Value=x0  SampleTime=TimeStep
  iniVEHposition wrtGLOB [m]1 : Constant  Value=y0  SampleTime=TimeStep
  iniVEHposition wrtGLOB [m]2 : Constant  Value=z0  SampleTime=TimeStep
  state2FullState : PreScanSimulinkLibrary/state2FullState  SystemSampleTime=-1
  StateBus : Outport  OutDataTypeStr=Bus: PRESCAN_STATEACTUATORDATA
  wires:
  Mux2/1 -> state2FullState/4
  iniVEHAngles wrtGLOB [rad]/1 -> Mux2/3
  Mux1/1 -> state2FullState/3
  Constant/1 -> Mux2/1, Mux2/2, Mux1/3
  iniBODYAngles wrtVEH [rad]1/1 -> Mux1/2
  iniBODYAngles wrtVEH [rad]/1 -> Mux1/1
  Mux/1 -> state2FullState/2
  iniVEHposition wrtGLOB [m]2/1 -> Mux/3
  iniVEHposition wrtGLOB [m]/1 -> Mux/1
  iniVEHposition wrtGLOB [m]1/1 -> Mux/2
  Demux/15 -> Bus Creator/15  "AngularVelocityYaw"
  Demux/14 -> Bus Creator/14  "AngularVelocityPitch"
  Demux/13 -> Bus Creator/13  "AngularVelocityRoll"
  Demux/12 -> Bus Creator/12  "OrientationYaw"
  Demux/11 -> Bus Creator/11  "OrientationPitch"
  Demux/10 -> Bus Creator/10  "OrientationRoll"
  Demux/9 -> Bus Creator/9  "AccelerationZ"
  Demux/8 -> Bus Creator/8  "AccelerationY"
  Demux/7 -> Bus Creator/7  "AccelerationX"
  Demux/6 -> Bus Creator/6  "VelocityZ"
  Demux/5 -> Bus Creator/5  "VelocityY"
  Demux/4 -> Bus Creator/4  "VelocityX"
  Demux/3 -> Bus Creator/3  "PositionZ"
  Demux/2 -> Bus Creator/2  "PositionY"
  Demux/1 -> Bus Creator/1  "PositionX"
  state2FullState/1 -> Demux/1
  State/1 -> state2FullState/1
  Bus Creator/1 -> StateBus/1

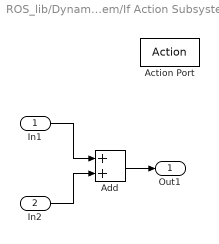
== system ROS_lib/Dynamics_Empty/Subsystem/If Action Subsystem ==
  In1 : Inport
  In2 : Inport  Port=2
  Action Port : ActionPort
  Add : Sum
  Out1 : Outport
  wires:
  In2/1 -> Add/2
  In1/1 -> Add/1
  Add/1 -> Out1/1

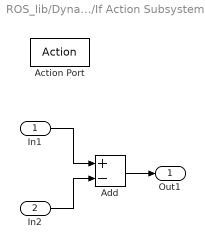
== system ROS_lib/Dynamics_Empty/Subsystem/If Action Subsystem1 ==
  In1 : Inport
  In2 : Inport  Port=2
  Action Port : ActionPort
  Add : Sum  Inputs=+-
  Out1 : Outport
  wires:
  In1/1 -> Add/1
  In2/1 -> Add/2
  Add/1 -> Out1/1

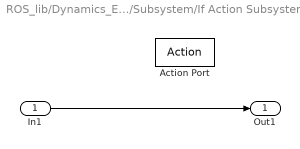
== system ROS_lib/Dynamics_Empty/Subsystem/If Action Subsystem2 ==
  In1 : Inport
  Action Port : ActionPort
  Out1 : Outport
  wires:
  In1/1 -> Out1/1
